simulink model "DC_motor_Generator_set"  (R2020a)
settings: Solver=VariableStepAuto  StartTime=0.0  StopTime=10.0  RelTol=1e-3
InitFcn:
  | Va=240;
  | Vf=5;
  | 
  | Rf=5;
  | Maf=1.8;
  | Lf=2;
  | J=.086;
  | B=0;
  | La=10.4*10^-3;
  | Ra=1.43;
  | 
  | Rf1=5;
  | Kv1=1.8;
  | Maf1=1.8;
  | If1=Kv1/Maf1;
  | Vf1=If1*Rf1;
  | Lf1=.2;
  | J1=.086;
  | B1=0;
  | La1=10.4*10^(-3);
  | Ra1=1.43;
  | L1=10.4*10^-3;
  | Ra1=1.43;
settings Model: Creator=User  LastModifiedBy=User

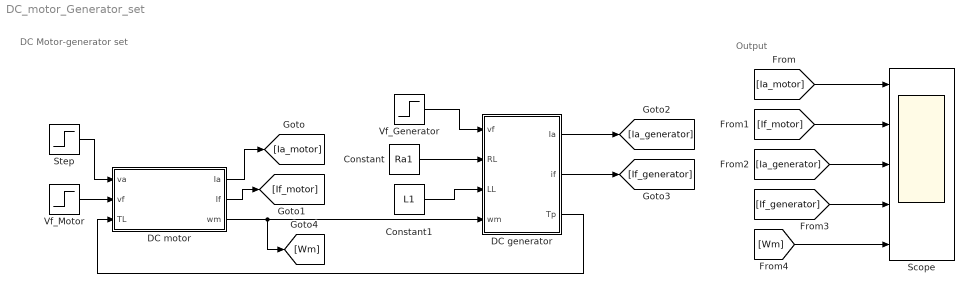
== system DC_motor_Generator_set ==
  note: DC Motor-generator set
  note: Output
  Constant : Constant  Value=Ra1
  Constant1 : Constant  Value=L1
  DC generator : Subsystem
  DC motor : Subsystem
  Scope : Scope  NumInputPorts=5
  Step : Step  After=Va  SampleTime=0
  Vf_Generator : Step  Before=Vf1  After=Vf1  SampleTime=0
  Vf_Motor : Step  Before=Vf  After=Vf  SampleTime=0
  wires:
  DC motor/3(wm) -> [Wm], DC generator/4(wm)
  Constant1/1 -> DC generator/3(LL)
  Constant/1 -> DC generator/2(RL)
  DC generator/3(Tp) -> DC motor/3(TL)
  Vf_Motor/1 -> DC motor/2(vf)
  Step/1 -> DC motor/1(va)
  Vf_Generator/1 -> DC generator/1(vf)
  DC motor/2(If) -> [If_motor]
  DC motor/1(Ia) -> [Ia_motor]
  DC generator/1(Ia) -> [Ia_generator]
  DC generator/2(if) -> [If_generator]
  [Ia_motor] -> Scope/1
  [If_motor] -> Scope/2
  [Ia_generator] -> Scope/3
  [If_generator] -> Scope/4
  [Wm] -> Scope/5

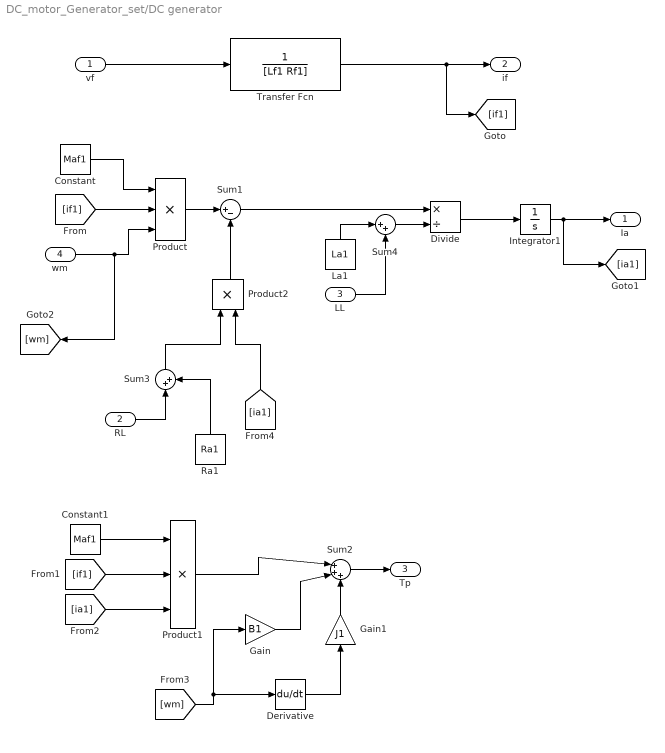
== system DC_motor_Generator_set/DC generator ==
  vf : Inport
  RL : Inport  Port=2
  LL : Inport  Port=3
  wm : Inport  Port=4
  Constant : Constant  Value=Maf1
  Constant1 : Constant  Value=Maf1
  Derivative : Derivative
  Divide : Product  Inputs=*/
  Gain : Gain  Gain=B1
  Gain1 : Gain  Gain=J1
  Integrator1 : Integrator
  La1 : Constant  Value=La1
  Product : Product  Inputs=3
  Product1 : Product  Inputs=3
  Product2 : Product
  Ra1 : Constant  Value=Ra1
  Sum1 : Sum  Inputs=|+-
  Sum2 : Sum  Inputs=|+++
  Sum3 : Sum  Inputs=|++
  Sum4 : Sum  Inputs=|++
  Transfer Fcn : TransferFcn  Denominator=[Lf1 Rf1]
  Ia : Outport
  if : Outport  Port=2
  Tp : Outport  Port=3
  wires:
  [if1] -> Product/2
  vf/1 -> Transfer Fcn/1
  Constant/1 -> Product/1
  Constant1/1 -> Product1/1
  wm/1 -> [wm], Product/3
  Product/1 -> Sum1/1
  Product1/1 -> Sum2/1
  [if1] -> Product1/2
  [ia1] -> Product1/3
  RL/1 -> Sum3/1
  Ra1/1 -> Sum3/2
  LL/1 -> Sum4/2
  La1/1 -> Sum4/1
  Sum1/1 -> Divide/1
  Sum4/1 -> Divide/2
  Divide/1 -> Integrator1/1
  Integrator1/1 -> Ia/1, [ia1]
  Product2/1 -> Sum1/2
  Sum3/1 -> Product2/1
  [ia1] -> Product2/2
  Transfer Fcn/1 -> [if1], if/1
  [wm] -> Derivative/1, Gain/1
  Gain/1 -> Sum2/2
  Gain1/1 -> Sum2/3
  Derivative/1 -> Gain1/1
  Sum2/1 -> Tp/1

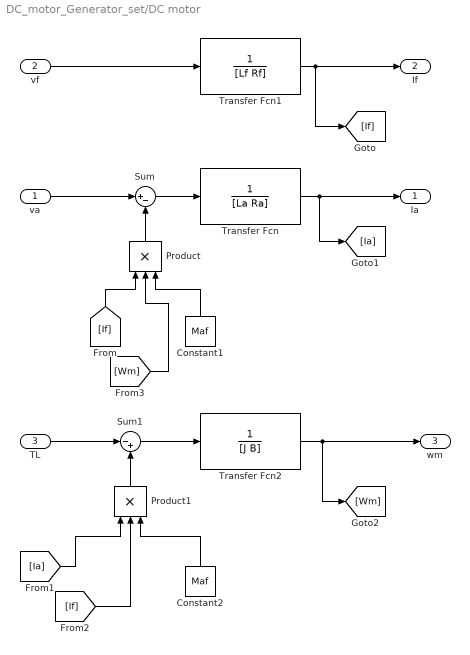
== system DC_motor_Generator_set/DC motor ==
  va : Inport
  vf : Inport  Port=2
  TL : Inport  Port=3
  Constant1 : Constant  Value=Maf
  Constant2 : Constant  Value=Maf
  Product : Product  Inputs=3
  Product1 : Product  Inputs=3
  Sum : Sum  Inputs=|+-
  Sum1 : Sum  Inputs=|-+
  Transfer Fcn : TransferFcn  Denominator=[La Ra]
  Transfer Fcn1 : TransferFcn  Denominator=[Lf Rf]
  Transfer Fcn2 : TransferFcn  Denominator=[J B]
  Ia : Outport
  If : Outport  Port=2
  wm : Outport  Port=3
  wires:
  Transfer Fcn/1 -> Ia/1, [Ia]
  Product1/1 -> Sum1/2
  vf/1 -> Transfer Fcn1/1
  Product/1 -> Sum/2
  Sum1/1 -> Transfer Fcn2/1
  Transfer Fcn1/1 -> If/1, [If]
  Transfer Fcn2/1 -> wm/1, [Wm]
  va/1 -> Sum/1
  Sum/1 -> Transfer Fcn/1
  [Ia] -> Product1/1
  [Wm] -> Product/2
  [If] -> Product1/2
  TL/1 -> Sum1/1
  [If] -> Product/1
  Constant2/1 -> Product1/3
  Constant1/1 -> Product/3
